simulink model "ik_omni"  (R2015a)
settings: Solver=ode45  StartTime=0.0  StopTime=10.0  RelTol=1e-3
libraries: aerolibutil x2
settings Model: Creator=Pinnacle  LastModifiedBy=Pinnacle

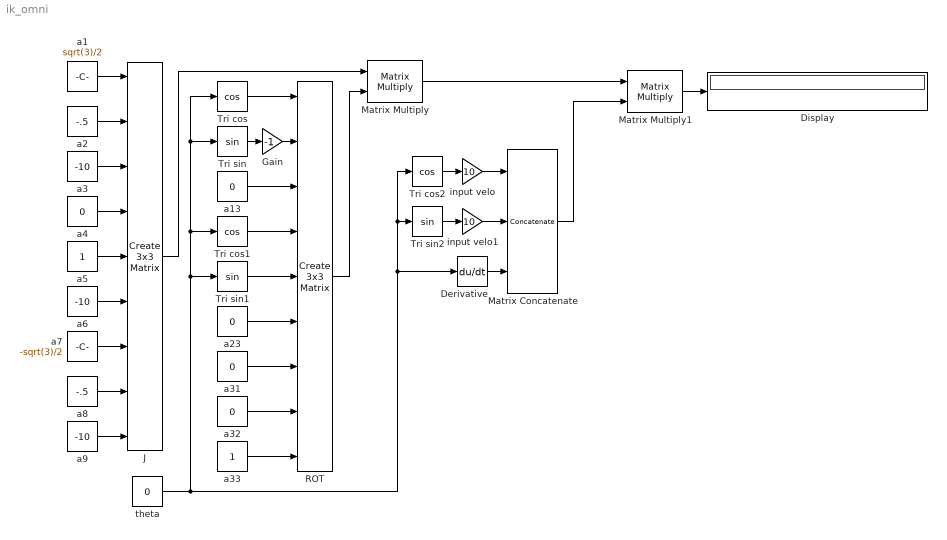
== system ik_omni ==
  Derivative : Derivative
  Display : Display
  Gain : Gain  Gain=-1
  J : aerolibutil/Create 3x3 Matrix
  Matrix Concatenate : Concatenate  NumInputs=3  Mode=Multidimensional array
  Matrix Multiply : Product  Multiplication=Matrix(*)
  Matrix Multiply1 : Product  Multiplication=Matrix(*)
  ROT : aerolibutil/Create 3x3 Matrix
  Tri cos : Trigonometry  Operator=cos
  Tri cos1 : Trigonometry  Operator=cos
  Tri cos2 : Trigonometry  Operator=cos
  Tri sin : Trigonometry
  Tri sin1 : Trigonometry
  Tri sin2 : Trigonometry
  a1 : Constant  Value=sqrt(3)/2
  a{4,13,23,31..32} (5 alike) : Constant  Value=0
  a2 : Constant  Value=-.5
  a3 : Constant  Value=-10
  a33 : Constant
  a5 : Constant
  a6 : Constant  Value=-10
  a7 : Constant  Value=-sqrt(3)/2
  a8 : Constant  Value=-.5
  a9 : Constant  Value=-10
  input velo : Gain  Gain=10
  input velo1 : Gain  Gain=10
  theta : Constant  Value=0
  wires:
  Tri cos/1 -> ROT/1
  a13/1 -> ROT/3
  Tri cos1/1 -> ROT/4
  Tri sin1/1 -> ROT/5
  a23/1 -> ROT/6
  a31/1 -> ROT/7
  a32/1 -> ROT/8
  a33/1 -> ROT/9
  Tri sin/1 -> Gain/1
  Gain/1 -> ROT/2
  a2/1 -> J/2
  a4/1 -> J/4
  a1/1 -> J/1
  a3/1 -> J/3
  a5/1 -> J/5
  a6/1 -> J/6
  a7/1 -> J/7
  a8/1 -> J/8
  a9/1 -> J/9
  Derivative/1 -> Matrix Concatenate/3
  J/1 -> Matrix Multiply/1
  ROT/1 -> Matrix Multiply/2
  Matrix Multiply/1 -> Matrix Multiply1/1
  Matrix Concatenate/1 -> Matrix Multiply1/2
  input velo/1 -> Matrix Concatenate/1
  Tri cos2/1 -> input velo/1
  Tri sin2/1 -> input velo1/1
  input velo1/1 -> Matrix Concatenate/2
  theta/1 -> Tri sin1/1, Tri cos1/1, Tri sin/1, Tri cos/1, Tri sin2/1, Tri cos2/1, Derivative/1
  Matrix Multiply1/1 -> Display/1
